simulink model "Boeing787_NewMission_ElectricalThermalHydraulicECS"  (R2016a)
settings: Solver=ode23tb  SolverMode=SingleTasking  StartTime=0.0  StopTime=346  RelTol=1e-3
InitFcn:
  | load('SampleOutput.mat')
  | 
  | load('SampleFuelBurn.mat')
undefined symbols (not defined in the file): ailerons, AirProp, B_737, CurrentMission, elevator, FuelBurn, HydProp, landing_gear, rudder, seed, thrust_rev
libraries: PowerFlowLib x68, simulink x20, powerlib_meascontrol x1
(part 14 of 24)

== system Boeing787_NewMission_ElectricalThermalHydraulicECS/Electrical/Generation Unit Sync-Sync4 ==
  engine speed : Inport
  battery voltage : Inport  Port=2
  idq0 : Inport  Port=3
  Temperature : Inport  Port=4
  Bus Creator : BusCreator  Inputs=3
  Bus Creator1 : BusCreator  Inputs=3
  Chopper (Averaged) : Subsystem  mask(Chopper.){}
      mask help: Basic chopper. Lossless storage elements. Switching model.
  Coeff of Resistance : Gain  Gain=3.85e-3
  Demux : Demux  Outputs=3
  Dot Product : DotProduct  InputSameDT=on  OutDataTypeStr=Inherit: Inherit via internal rule
  Exciter : Subsystem
      mask Display:
      | p = 0:0.1:(2*pi+0.1);
      | plot(sin(p), cos(p));
      | p1 = (-pi/8-0.1-0.2):0.1:(pi/8+0.1-0.2);
      | plot(0.8*sin(p1), 0.8*cos(p1), 0.8*sin(p1+pi), 0.8*cos(p1+pi));
      | p2 = sin((-pi/8-0.1-0.2+pi/8+0.1-0.2)/2);
      | p3 = sin((-pi/8-0.1-0.2+pi/8+0.1-0.2)/2+pi);
      | p4 = cos((-pi/8-0.1-0.2+pi/8+0.1-0.2)/2);
      | p5 = cos((-pi/8-0.1-0.2+pi/8+0.1-0.2)/2+pi);
      | plot(0.8*[p2, p3], 0.8*[p4, p5]);
      | port_label('output', 1, 'Vdq0');
      | port_label('output', 2, 'Te');
      | port_label('output', 3, 'Vfd');
      | port_label('output', 4, 'Ploss');
      | port_label('input', 1, 'idq0');
      | port_label('input', 2, 'w');
      | port_label('input', 3, 'ifd');
  Gain : Gain  Gain=200*2/3
  Gain1 : Gain  Gain=200
  Gain4 : Gain  Gain=0.001
  Gain5 : Gain  Gain=30
  Gain6 : Gain  Gain=0.02
  Generator : Subsystem
      mask Display:
      | p = 0:0.1:(2*pi+0.1);
      | plot(sin(p), cos(p));
      | p1 = (-pi/8-0.1-0.2):0.1:(pi/8+0.1-0.2);
      | plot(0.8*sin(p1), 0.8*cos(p1), 0.8*sin(p1+pi), 0.8*cos(p1+pi));
      | p2 = sin((-pi/8-0.1-0.2+pi/8+0.1-0.2)/2);
      | p3 = sin((-pi/8-0.1-0.2+pi/8+0.1-0.2)/2+pi);
      | p4 = cos((-pi/8-0.1-0.2+pi/8+0.1-0.2)/2);
      | p5 = cos((-pi/8-0.1-0.2+pi/8+0.1-0.2)/2+pi);
      | plot(0.8*[p2, p3], 0.8*[p4, p5]);
      | port_label('output', 1, 'Vdq0');
      | port_label('output', 2, 'Te');
      | port_label('output', 3, 'Vfd');
      | port_label('output', 4, 'Ploss');
      | port_label('input', 1, 'idq0');
      | port_label('input', 2, 'w');
      | port_label('input', 3, 'ifd');
  Initial Temperature : Constant  Value=25
  Integrator : Integrator  LimitOutput=on  UpperSaturationLimit=10  LowerSaturationLimit=-10
  Integrator1 : Integrator  LimitOutput=on  UpperSaturationLimit=1  LowerSaturationLimit=0
  RPM_to_radps : Gain  Gain=pi/30
  Sqrt : Sqrt  SaturateOnIntegerOverflow=on
  Sum : Sum  Inputs=++|
  Sum1 : Sum
  Sum2 : Sum  Inputs=+-|
  Sum3 : Sum  Inputs=-+|
  Sum4 : Sum  Inputs=+
  Sum5 : Sum  Inputs=|+-
  Sum6 : Sum  Inputs=|++
  Vcmd : Constant  Value=Vnom
  control1 : Constant
  data_sink : PowerFlowLib/Support Functions//Tools/data_sink
  one : Constant
  three-phase active rectifier Voltage Mode : PowerFlowLib/Energy & Power Systems/Electrical/Rectifiers/three-phase  active rectifier Voltage Mode  L=1  C=1e-4
  vdq0 : Outport
  battery current : Outport  Port=2
  engine torque : Outport  Port=3
  Ploss : Outport  Port=4
  wires:
  [R_temp_delta] -> Generator/4(Temp)
  [R_temp_delta] -> Exciter/4(Temp)
  [R_temp_delta] -> Chopper (Averaged)/3(Temperature)
  Sum6/1 -> [R_temp_delta]
  one/1 -> Sum6/2
  Coeff of Resistance/1 -> Sum6/1
  Sum5/1 -> Coeff of Resistance/1
  Initial Temperature/1 -> Sum5/2
  Temperature/1 -> Sum5/1
  engine speed/1 -> RPM_to_radps/1
  Bus Creator1/1 -> Bus Creator/1  "vdq0 (V)"
  Demux/3 -> Bus Creator1/3  "v0"
  Demux/2 -> Bus Creator1/2  "vq"
  Demux/1 -> Bus Creator1/1  "vd"
  Bus Creator/1 -> data_sink/1
  Sum/1 -> engine torque/1
  RPM_to_radps/1 -> Exciter/2(w), Generator/2(w)
  Exciter/1(vdq0) -> three-phase active rectifier Voltage Mode/1
  control1/1 -> three-phase active rectifier Voltage Mode/2
  Generator/3(vfd') -> Gain1/1
  Gain1/1 -> three-phase active rectifier Voltage Mode/3
  Gain/1 -> Bus Creator/3, Generator/3(ifd')  "Exciter current (A)"
  three-phase active rectifier Voltage Mode/1 -> Gain/1
  Exciter/2(Te) -> Sum/1
  Generator/2(Te) -> Sum/2
  idq0/1 -> Generator/1(idq0)
  Generator/1(vdq0) -> Demux/1, vdq0/1, Dot Product/2, Dot Product/1  "Vdq0 (V)"
  Chopper (Averaged)/1(iout) -> Exciter/3(ifd')
  battery voltage/1 -> Chopper (Averaged)/1(vin)
  Chopper (Averaged)/2(iin) -> battery current/1
  Exciter/4(Ploss) -> Sum1/1
  Generator/4(Ploss) -> Sum1/2
  Sum1/1 -> Ploss/1, Bus Creator/2  "Ploss (W)"
  Gain4/1 -> Integrator/1
  Sum2/1 -> Gain4/1
  Integrator/1 -> Sum3/2
  Sum3/1 -> Gain6/1
  Vcmd/1 -> Sum2/1
  Dot Product/1 -> Sum4/1
  Sum4/1 -> Sqrt/1
  Sqrt/1 -> Sum2/2
  Gain6/1 -> Integrator1/1
  Gain5/1 -> Sum3/1
  three-phase active rectifier Voltage Mode/2 -> Exciter/1(idq0)
  Integrator1/1 -> Chopper (Averaged)/2(q), Gain5/1

== system Boeing787_NewMission_ElectricalThermalHydraulicECS/Electrical/Generation Unit Sync-Sync5 ==
  engine speed : Inport
  battery voltage : Inport  Port=2
  idq0 : Inport  Port=3
  Temperature : Inport  Port=4
  Bus Creator : BusCreator  Inputs=3
  Bus Creator1 : BusCreator  Inputs=3
  Chopper (Averaged) : Subsystem  mask(Chopper.){}
      mask help: Basic chopper. Lossless storage elements. Switching model.
  Coeff of Resistance : Gain  Gain=3.85e-3
  Demux : Demux  Outputs=3
  Dot Product : DotProduct  InputSameDT=on  OutDataTypeStr=Inherit: Inherit via internal rule
  Exciter : Subsystem
      mask Display:
      | p = 0:0.1:(2*pi+0.1);
      | plot(sin(p), cos(p));
      | p1 = (-pi/8-0.1-0.2):0.1:(pi/8+0.1-0.2);
      | plot(0.8*sin(p1), 0.8*cos(p1), 0.8*sin(p1+pi), 0.8*cos(p1+pi));
      | p2 = sin((-pi/8-0.1-0.2+pi/8+0.1-0.2)/2);
      | p3 = sin((-pi/8-0.1-0.2+pi/8+0.1-0.2)/2+pi);
      | p4 = cos((-pi/8-0.1-0.2+pi/8+0.1-0.2)/2);
      | p5 = cos((-pi/8-0.1-0.2+pi/8+0.1-0.2)/2+pi);
      | plot(0.8*[p2, p3], 0.8*[p4, p5]);
      | port_label('output', 1, 'Vdq0');
      | port_label('output', 2, 'Te');
      | port_label('output', 3, 'Vfd');
      | port_label('output', 4, 'Ploss');
      | port_label('input', 1, 'idq0');
      | port_label('input', 2, 'w');
      | port_label('input', 3, 'ifd');
  Gain : Gain  Gain=200*2/3
  Gain1 : Gain  Gain=200
  Gain4 : Gain  Gain=0.001
  Gain5 : Gain  Gain=30
  Gain6 : Gain  Gain=0.02
  Generator : Subsystem
      mask Display:
      | p = 0:0.1:(2*pi+0.1);
      | plot(sin(p), cos(p));
      | p1 = (-pi/8-0.1-0.2):0.1:(pi/8+0.1-0.2);
      | plot(0.8*sin(p1), 0.8*cos(p1), 0.8*sin(p1+pi), 0.8*cos(p1+pi));
      | p2 = sin((-pi/8-0.1-0.2+pi/8+0.1-0.2)/2);
      | p3 = sin((-pi/8-0.1-0.2+pi/8+0.1-0.2)/2+pi);
      | p4 = cos((-pi/8-0.1-0.2+pi/8+0.1-0.2)/2);
      | p5 = cos((-pi/8-0.1-0.2+pi/8+0.1-0.2)/2+pi);
      | plot(0.8*[p2, p3], 0.8*[p4, p5]);
      | port_label('output', 1, 'Vdq0');
      | port_label('output', 2, 'Te');
      | port_label('output', 3, 'Vfd');
      | port_label('output', 4, 'Ploss');
      | port_label('input', 1, 'idq0');
      | port_label('input', 2, 'w');
      | port_label('input', 3, 'ifd');
  Initial Temperature : Constant  Value=25
  Integrator : Integrator  LimitOutput=on  UpperSaturationLimit=10  LowerSaturationLimit=-10
  Integrator1 : Integrator  LimitOutput=on  UpperSaturationLimit=1  LowerSaturationLimit=0
  RPM_to_radps : Gain  Gain=pi/30
  Sqrt : Sqrt  SaturateOnIntegerOverflow=on
  Sum : Sum  Inputs=++|
  Sum1 : Sum
  Sum2 : Sum  Inputs=+-|
  Sum3 : Sum  Inputs=-+|
  Sum4 : Sum  Inputs=+
  Sum5 : Sum  Inputs=|+-
  Sum6 : Sum  Inputs=|++
  Vcmd : Constant  Value=Vnom
  control1 : Constant
  data_sink : PowerFlowLib/Support Functions//Tools/data_sink
  one : Constant
  three-phase active rectifier Voltage Mode : PowerFlowLib/Energy & Power Systems/Electrical/Rectifiers/three-phase  active rectifier Voltage Mode  L=1  C=1e-4
  vdq0 : Outport
  battery current : Outport  Port=2
  engine torque : Outport  Port=3
  Ploss : Outport  Port=4
  wires:
  Integrator1/1 -> Gain5/1, Chopper (Averaged)/2(q)
  three-phase active rectifier Voltage Mode/2 -> Exciter/1(idq0)
  Gain5/1 -> Sum3/1
  Gain6/1 -> Integrator1/1
  Sqrt/1 -> Sum2/2
  Sum4/1 -> Sqrt/1
  Dot Product/1 -> Sum4/1
  Vcmd/1 -> Sum2/1
  Sum3/1 -> Gain6/1
  Integrator/1 -> Sum3/2
  Sum2/1 -> Gain4/1
  Gain4/1 -> Integrator/1
  Sum1/1 -> Bus Creator/2, Ploss/1  "Ploss (W)"
  Generator/4(Ploss) -> Sum1/2
  Exciter/4(Ploss) -> Sum1/1
  Chopper (Averaged)/2(iin) -> battery current/1
  battery voltage/1 -> Chopper (Averaged)/1(vin)
  Chopper (Averaged)/1(iout) -> Exciter/3(ifd')
  Generator/1(vdq0) -> Dot Product/1, Dot Product/2, vdq0/1, Demux/1  "Vdq0 (V)"
  idq0/1 -> Generator/1(idq0)
  Generator/2(Te) -> Sum/2
  Exciter/2(Te) -> Sum/1
  three-phase active rectifier Voltage Mode/1 -> Gain/1
  Gain/1 -> Generator/3(ifd'), Bus Creator/3  "Exciter current (A)"
  Gain1/1 -> three-phase active rectifier Voltage Mode/3
  Generator/3(vfd') -> Gain1/1
  control1/1 -> three-phase active rectifier Voltage Mode/2
  Exciter/1(vdq0) -> three-phase active rectifier Voltage Mode/1
  RPM_to_radps/1 -> Generator/2(w), Exciter/2(w)
  Sum/1 -> engine torque/1
  Bus Creator/1 -> data_sink/1
  Demux/1 -> Bus Creator1/1  "vd"
  Demux/2 -> Bus Creator1/2  "vq"
  Demux/3 -> Bus Creator1/3  "v0"
  Bus Creator1/1 -> Bus Creator/1  "vdq0 (V)"
  engine speed/1 -> RPM_to_radps/1
  Temperature/1 -> Sum5/1
  Initial Temperature/1 -> Sum5/2
  Sum5/1 -> Coeff of Resistance/1
  Coeff of Resistance/1 -> Sum6/1
  one/1 -> Sum6/2
  Sum6/1 -> [R_temp_delta]
  [R_temp_delta] -> Chopper (Averaged)/3(Temperature)
  [R_temp_delta] -> Exciter/4(Temp)
  [R_temp_delta] -> Generator/4(Temp)

== system Boeing787_NewMission_ElectricalThermalHydraulicECS/Electrical/Loads ==
  115VAC : Lookup_n-D  NumberOfTableDimensions=1  BreakpointsForDimension1=CurrentMission.tvec  Table=CurrentMission.V115ac  InterpMethod=Flat  InternalRulePriority=Speed  RndMeth=Simplest  InputSameDT=on
  230VAC : Lookup_n-D  NumberOfTableDimensions=1  BreakpointsForDimension1=CurrentMission.tvec  Table=CurrentMission.V230ac  InterpMethod=Flat  InternalRulePriority=Speed  RndMeth=Simplest  InputSameDT=on
  270VDC : Lookup_n-D  NumberOfTableDimensions=1  BreakpointsForDimension1=CurrentMission.tvec  Table=CurrentMission.V270dc  InterpMethod=Flat  InternalRulePriority=Speed  RndMeth=Simplest  InputSameDT=on
  28VDC : Lookup_n-D  NumberOfTableDimensions=1  BreakpointsForDimension1=CurrentMission.tvec  Table=CurrentMission.V28dc  InterpMethod=Flat  InternalRulePriority=Speed  RndMeth=Simplest  InputSameDT=on
  Clock : Clock
  Constant{,1..3} (4 alike) : Constant  Value=0
  Mux{,1..3} (4 alike) : Mux  Inputs=3
  PF{1..4} (4 alike) : Gain  Gain=0
  Product{,1..3} (4 alike) : Product
  Uniform Random Number : UniformRandomNumber  Minimum=0.95  Maximum=1.05  Seed=seed+500  SampleTime=1
  Uniform Random Number1 : UniformRandomNumber  Minimum=0.95  Maximum=1.05  Seed=seed  SampleTime=1
  Uniform Random Number2 : UniformRandomNumber  Minimum=0.95  Maximum=1.05  SampleTime=1
  Uniform Random Number3 : UniformRandomNumber  Minimum=0.95  Maximum=1.05  SampleTime=1
  kW to W{,1..3} (4 alike) : Gain  Gain=1000
  230 Vac Loads : Outport
  115 Vac Loads : Outport  Port=2
  270 Vdc Loads : Outport  Port=3
  28 Vdc Loads : Outport  Port=4
  wires:
  Mux2/1 -> 230 Vac Loads/1
  Mux/1 -> 270 Vdc Loads/1
  Clock/1 -> 28VDC/1, 270VDC/1, 115VAC/1, 230VAC/1
  PF3/1 -> Mux/2  "Q"
  270VDC/1 -> kW to W1/1  "P"
  PF2/1 -> Mux1/2  "Q"
  115VAC/1 -> kW to W2/1  "P"
  PF1/1 -> Mux2/2  "Q"
  230VAC/1 -> kW to W/1  "P"
  PF4/1 -> Mux3/2  "Q"
  28VDC/1 -> kW to W3/1  "P"
  Mux3/1 -> 28 Vdc Loads/1
  Constant/1 -> Mux/3
  Constant1/1 -> Mux3/3
  Constant2/1 -> Mux1/3
  Constant3/1 -> Mux2/3
  Mux1/1 -> 115 Vac Loads/1
  Product1/1 -> PF1/1, Mux2/1
  Product/1 -> PF2/1, Mux1/1
  Product2/1 -> PF3/1, Mux/1
  Product3/1 -> PF4/1, Mux3/1
  kW to W2/1 -> Product/2
  kW to W/1 -> Product1/2
  kW to W1/1 -> Product2/2
  kW to W3/1 -> Product3/2
  Uniform Random Number3/1 -> Product3/1
  Uniform Random Number2/1 -> Product2/1
  Uniform Random Number1/1 -> Product1/1
  Uniform Random Number/1 -> Product/1

== system Boeing787_NewMission_ElectricalThermalHydraulicECS/Electrical/Outputs ==
  Left_Wing_Toqrue_Nm : Inport
  Rght_Wing_Torque_Nm : Inport  Port=2
  APU_Torque_Nm : Inport  Port=3
  DC_Voltage_270 : Inport  Port=4
  Bus Creator : BusCreator  Inputs=4
  Electrical : Outport
  wires:
  Rght_Wing_Torque_Nm/1 -> Bus Creator/2  "Right Wing Torq (Nm)"
  APU_Torque_Nm/1 -> Bus Creator/3  "APU Torq (Nm)"
  Left_Wing_Toqrue_Nm/1 -> Bus Creator/1  "Left Wing Torq (Nm)"
  Bus Creator/1 -> Electrical/1
  DC_Voltage_270/1 -> Bus Creator/4  "DC_Voltage_270"

== system Boeing787_NewMission_ElectricalThermalHydraulicECS/Electrical/Thermal Interface ==
  Generator Loss [4] : Inport
  APU Loss [2] : Inport  Port=2
  Battery Loss [1] : Inport  Port=3
  Loadloss_W : Inport  Port=4
  Battery Thermal Model : Subsystem
  Constant{,1,3..4} (4 alike) : Constant  Value=0
  Constant2 : Constant  Value=25
  Constant5 : Constant  Value=25
  Coolant Temp : Constant  Value=25
  Coolant mdot : Constant  Value=0.5
  Demux : Demux
  Demux1 : Demux  Outputs=2
  Gain : Gain  Gain=50
  Generator 1 Thermal Model : Subsystem
  Generator 2 Thermal Model : Subsystem
  Generator 3 Thermal Model : Subsystem
  Generator 4 Thermal Model : Subsystem
  Generator 5 Thermal Model : Subsystem
  Generator 6 Thermal Model : Subsystem
  Load Thermal Model : Subsystem
  Mux : Mux
  To Workspace6 : ToWorkspace  VariableName=gen_temps  SaveFormat=Structure With Time  SampleTime=-1
  air Temp : Constant  Value=25
  Tgen1 : Outport
  Tgen2 : Outport  Port=2
  Tgen3 : Outport  Port=3
  Tgen4 : Outport  Port=4
  Tgen5 : Outport  Port=5
  Tgen6 : Outport  Port=6
  Tbatt : Outport  Port=7
  TLoad : Outport  Port=8
  wires:
  Generator Loss [4]/1 -> Gain/1
  Demux/1 -> Generator 1 Thermal Model/1(Ploss)
  Demux/2 -> Generator 2 Thermal Model/1(Ploss)
  Demux/3 -> Generator 3 Thermal Model/1(Ploss)
  Demux/4 -> Generator 4 Thermal Model/1(Ploss)
  Generator 4 Thermal Model/1(T_gen) -> Mux/4, Tgen4/1
  Generator 2 Thermal Model/1(T_gen) -> Mux/2, Tgen2/1
  Generator 1 Thermal Model/1(T_gen) -> Mux/1, Tgen1/1
  APU Loss [2]/1 -> Demux1/1
  Demux1/1 -> Generator 5 Thermal Model/1(Ploss)
  Demux1/2 -> Generator 6 Thermal Model/1(Ploss)
  Generator 6 Thermal Model/1(T_gen) -> Tgen6/1
  Generator 5 Thermal Model/1(T_gen) -> Tgen5/1
  Coolant Temp/1 -> [Tf]
  air Temp/1 -> [Ta]
  Coolant mdot/1 -> [mdot]
  [mdot] -> Generator 1 Thermal Model/4(coolant mdot)
  [Tf] -> Generator 1 Thermal Model/2(Liquid Coolant Temp)
  [Ta] -> Generator 1 Thermal Model/3(Air Temp)
  [Tf] -> Generator 6 Thermal Model/2(Liquid Coolant Temp)
  [Ta] -> Generator 6 Thermal Model/3(Air Temp)
  [mdot] -> Generator 6 Thermal Model/4(coolant mdot)
  [Tf] -> Generator 5 Thermal Model/2(Liquid Coolant Temp)
  [Ta] -> Generator 5 Thermal Model/3(Air Temp)
  [mdot] -> Generator 5 Thermal Model/4(coolant mdot)
  [mdot] -> Generator 4 Thermal Model/4(coolant mdot)
  [Ta] -> Generator 4 Thermal Model/3(Air Temp)
  [Tf] -> Generator 4 Thermal Model/2(Liquid Coolant Temp)
  [Tf] -> Generator 3 Thermal Model/2(Liquid Coolant Temp)
  [Ta] -> Generator 3 Thermal Model/3(Air Temp)
  [mdot] -> Generator 3 Thermal Model/4(coolant mdot)
  [Tf] -> Generator 2 Thermal Model/2(Liquid Coolant Temp)
  [mdot] -> Generator 2 Thermal Model/4(coolant mdot)
  [Ta] -> Generator 2 Thermal Model/3(Air Temp)
  Battery Loss [1]/1 -> Battery Thermal Model/1(Ploss)
  Loadloss_W/1 -> Load Thermal Model/1(Ploss)
  Constant/1 -> Battery Thermal Model/2(Liquid Coolant Temp)
  Constant1/1 -> Battery Thermal Model/4(coolant mdot)
  Constant2/1 -> Battery Thermal Model/3(Air Temp)
  Constant4/1 -> Load Thermal Model/4(coolant mdot)
  Constant3/1 -> Load Thermal Model/2(Liquid Coolant Temp)
  Constant5/1 -> Load Thermal Model/3(Air Temp)
  Battery Thermal Model/1(T_Batt) -> Tbatt/1
  Load Thermal Model/1(T_gen) -> TLoad/1
  Generator 3 Thermal Model/1(T_gen) -> Mux/3, Tgen3/1
  Mux/1 -> To Workspace6/1
  Gain/1 -> Demux/1

== system Boeing787_NewMission_ElectricalThermalHydraulicECS/Electrical/Transformer-rectifier ==
  vqd0 : Inport
  iDC : Inport  Port=2
  Constant1 : Constant  Value=270
  Constant2 : Constant  Value=1.0
  Control : Subsystem
  Sum1 : Sum  Inputs=|++
  Three-phase Full Bridge Rectifier : Subsystem  AncestorBlock=PowerFlowLib/Energy & Power Systems/Electrical/Rectifiers/Three-phase Full Bridge1  mask(Single-phase full bridge rectifier.){C=100e-6, Rc=1}
      mask prompts: C "Output capacitance (F):"; Rc "Circuit parasitic resistance (ohm):"
      mask help: Single-phase Full bridge rectifier. Lead resistance is added to make simulation possible.
  Transformer1 : Subsystem  AncestorBlock=PowerFlowLib/Energy & Power Systems/Electrical/Machines/Transformer  mask(Transformer){Rp=0.005, Rs=0.1, N1=400, N2=332*1.4}
      mask prompts: Rp "Primary Winding Resistance"; Rs "Secondary Winding Resistance"; N1 "Number of Turns in Primary"; N2 "Number of Turns in Secondary"
      mask help:
      | The user inputs and outputs are given below. Inputs to the model are:
      |
      | Block Inputs
      | #1: Primary voltage input [V]
      | #2: Secondary current input [A]
      |
      | Block Outputs
      | #1: Secondary voltage output [V]
      | #2: Primary current input [A]
      mask Help: eval('open(''Transformer Help.html'')');
      mask Display:
      | image(imread('Transformer.png'))
      | 
      | port_label('input',1,'{\bf V_i_n}','TexMode','on')
      | port_label('input',2,'{\bf I_o_u_t}','TexMode','on')
      | 
      | port_label('output',1,'{\bf V_o_u_t}','TexMode','on')
      | port_label('output',2,'{\bf I_i_n}','TexMode','on')
  vout : Outport
  iqd0 : Outport  Port=2
  wires:
  Transformer1/2(Iin) -> iqd0/1
  Transformer1/1(Vout) -> Three-phase Full Bridge Rectifier/2(vin)
  vqd0/1 -> Transformer1/1(Vin)
  Three-phase Full Bridge Rectifier/2(iin) -> Transformer1/2(Iout)
  iDC/1 -> Three-phase Full Bridge Rectifier/1(iout)
  Three-phase Full Bridge Rectifier/1(vout) -> Control/1(Vout), vout/1
  Constant1/1 -> Control/2(ref)
  Constant2/1 -> Sum1/1
  Control/1(u) -> Sum1/2
  Sum1/1 -> Three-phase Full Bridge Rectifier/3(u)

== system Boeing787_NewMission_ElectricalThermalHydraulicECS/Electrical/Transformer-rectifier1 ==
  vqd0 : Inport
  iDC : Inport  Port=2
  Constant : Constant
  Constant1 : Constant  Value=28
  Control : Subsystem
  Saturation : Saturate  UpperLimit=inf  LowerLimit=-inf
  Sum1 : Sum  Inputs=|++
  Three-phase Full Bridge1 : Subsystem  AncestorBlock=PowerFlowLib/Energy & Power Systems/Electrical/Rectifiers/Three-phase Full Bridge1  mask(Single-phase full bridge rectifier.){C=100e-6, Rc=1}
      mask prompts: C "Output capacitance (F):"; Rc "Circuit parasitic resistance (ohm):"
      mask help: Single-phase Full bridge rectifier. Lead resistance is added to make simulation possible.
  Transformer1 : Subsystem  AncestorBlock=PowerFlowLib/Energy & Power Systems/Electrical/Machines/Transformer  mask(Transformer){Rp=0.005, Rs=0.1, N1=400, N2=45}
      mask prompts: Rp "Primary Winding Resistance"; Rs "Secondary Winding Resistance"; N1 "Number of Turns in Primary"; N2 "Number of Turns in Secondary"
      mask help:
      | The user inputs and outputs are given below. Inputs to the model are:
      |
      | Block Inputs
      | #1: Primary voltage input [V]
      | #2: Secondary current input [A]
      |
      | Block Outputs
      | #1: Secondary voltage output [V]
      | #2: Primary current input [A]
      mask Help: eval('open(''Transformer Help.html'')');
      mask Display:
      | image(imread('Transformer.png'))
      | 
      | port_label('input',1,'{\bf V_i_n}','TexMode','on')
      | port_label('input',2,'{\bf I_o_u_t}','TexMode','on')
      | 
      | port_label('output',1,'{\bf V_o_u_t}','TexMode','on')
      | port_label('output',2,'{\bf I_i_n}','TexMode','on')
  vout : Outport
  iqd0 : Outport  Port=2
  wires:
  Three-phase Full Bridge1/1(vout) -> Control/1(Vout), vout/1
  iDC/1 -> Three-phase Full Bridge1/1(iout)
  Three-phase Full Bridge1/2(iin) -> Transformer1/2(Iout)
  vqd0/1 -> Transformer1/1(Vin)
  Transformer1/1(Vout) -> Three-phase Full Bridge1/2(vin)
  Transformer1/2(Iin) -> iqd0/1
  Constant1/1 -> Control/2(ref)
  Constant/1 -> Sum1/1
  Control/1(u) -> Sum1/2
  Sum1/1 -> Saturation/1
  Saturation/1 -> Three-phase Full Bridge1/3(u)

== system Boeing787_NewMission_ElectricalThermalHydraulicECS/Eng1/Gearbox ==
  w_engine : Inport
  T_gen : Inport  Port=2
  1-tran_efficiency : Gain  Gain=1-Gear_Efficiency/100  SaturateOnIntegerOverflow=on  OutDataTypeStr=Inherit: Same as input  ParamDataTypeStr=Inherit: Same as input
  Gain : Gain  Gain=Gear_Ratio
  Gain1 : Gain  Gain=Gear_Ratio
  Memory1 : Memory
  Sum : Sum  Inputs=-++  SaturateOnIntegerOverflow=on  InputSameDT=on  OutDataTypeStr=Inherit: Same as first input
  gear1 NL loss : Lookup  InputValues=[0;1000;2000;3000;4000;5000;6000]*2*pi/60  Table=[0;0.735;1.334;1.491;1.525;1.212;1.276]  SaturateOnIntegerOverflow=on
  tran_efficiency : Gain  Gain=Gear_Efficiency/4/100  SaturateOnIntegerOverflow=on  OutDataTypeStr=Inherit: Same as input  ParamDataTypeStr=Inherit: Same as input
  w_shaft : Outport
  T_shaft : Outport  Port=2
  wires:
  Gain/1 -> w_shaft/1
  Gain1/1 -> Memory1/1
  T_gen/1 -> Gain1/1, 1-tran_efficiency/1
  w_engine/1 -> Gain/1, gear1 NL loss/1
  gear1 NL loss/1 -> tran_efficiency/1
  Memory1/1 -> Sum/3
  1-tran_efficiency/1 -> Sum/2
  tran_efficiency/1 -> Sum/1
  Sum/1 -> T_shaft/1

== system Boeing787_NewMission_ElectricalThermalHydraulicECS/Eng1/Unit Conversion  ==
  Signal_in : Inport
  conv_fcn : Fcn  Expr=u(1)/745.69987
  Converted Signal Out : Outport
  wires:
  Signal_in/1 -> conv_fcn/1
  conv_fcn/1 -> Converted Signal Out/1

== system Boeing787_NewMission_ElectricalThermalHydraulicECS/Eng1/Unit Conversion 1 ==
  Signal_in : Inport
  conv_fcn : Fcn  Expr=u(1)/1.8
  Converted Signal Out : Outport
  wires:
  conv_fcn/1 -> Converted Signal Out/1
  Signal_in/1 -> conv_fcn/1

== system Boeing787_NewMission_ElectricalThermalHydraulicECS/Eng1/Unit Conversion 4 ==
  Signal_in : Inport
  conv_fcn : Fcn  Expr=u(1)/(1.450377e-1)
  Converted Signal Out : Outport
  wires:
  Signal_in/1 -> conv_fcn/1
  conv_fcn/1 -> Converted Signal Out/1

== system Boeing787_NewMission_ElectricalThermalHydraulicECS/Eng1/Unit Conversion 5 ==
  Signal_in : Inport
  conv_fcn : Fcn  Expr=u(1)*.45359237
  Converted Signal Out : Outport
  wires:
  Signal_in/1 -> conv_fcn/1
  conv_fcn/1 -> Converted Signal Out/1

== system Boeing787_NewMission_ElectricalThermalHydraulicECS/Eng2/Gearbox ==
  w_engine : Inport
  T_gen : Inport  Port=2
  1-tran_efficiency : Gain  Gain=1-Gear_Efficiency/100  SaturateOnIntegerOverflow=on  OutDataTypeStr=Inherit: Same as input  ParamDataTypeStr=Inherit: Same as input
  Gain : Gain  Gain=Gear_Ratio
  Gain1 : Gain  Gain=Gear_Ratio
  Memory1 : Memory
  Sum : Sum  Inputs=-++  SaturateOnIntegerOverflow=on  InputSameDT=on  OutDataTypeStr=Inherit: Same as first input
  gear1 NL loss : Lookup  InputValues=[0;1000;2000;3000;4000;5000;6000]*2*pi/60  Table=[0;0.735;1.334;1.491;1.525;1.212;1.276]  SaturateOnIntegerOverflow=on
  tran_efficiency : Gain  Gain=Gear_Efficiency/4/100  SaturateOnIntegerOverflow=on  OutDataTypeStr=Inherit: Same as input  ParamDataTypeStr=Inherit: Same as input
  w_shaft : Outport
  T_shaft : Outport  Port=2
  wires:
  Sum/1 -> T_shaft/1
  tran_efficiency/1 -> Sum/1
  1-tran_efficiency/1 -> Sum/2
  Memory1/1 -> Sum/3
  gear1 NL loss/1 -> tran_efficiency/1
  w_engine/1 -> gear1 NL loss/1, Gain/1
  T_gen/1 -> 1-tran_efficiency/1, Gain1/1
  Gain1/1 -> Memory1/1
  Gain/1 -> w_shaft/1

== system Boeing787_NewMission_ElectricalThermalHydraulicECS/Eng2/Unit Conversion  ==
  Signal_in : Inport
  conv_fcn : Fcn  Expr=u(1)/745.69987
  Converted Signal Out : Outport
  wires:
  conv_fcn/1 -> Converted Signal Out/1
  Signal_in/1 -> conv_fcn/1

== system Boeing787_NewMission_ElectricalThermalHydraulicECS/Eng2/Unit Conversion 1 ==
  Signal_in : Inport
  conv_fcn : Fcn  Expr=u(1)/1.8
  Converted Signal Out : Outport
  wires:
  Signal_in/1 -> conv_fcn/1
  conv_fcn/1 -> Converted Signal Out/1

== system Boeing787_NewMission_ElectricalThermalHydraulicECS/Eng2/Unit Conversion 4 ==
  Signal_in : Inport
  conv_fcn : Fcn  Expr=u(1)/(1.450377e-1)
  Converted Signal Out : Outport
  wires:
  conv_fcn/1 -> Converted Signal Out/1
  Signal_in/1 -> conv_fcn/1

== system Boeing787_NewMission_ElectricalThermalHydraulicECS/Eng2/Unit Conversion 5 ==
  Signal_in : Inport
  conv_fcn : Fcn  Expr=u(1)*.45359237
  Converted Signal Out : Outport
  wires:
  conv_fcn/1 -> Converted Signal Out/1
  Signal_in/1 -> conv_fcn/1

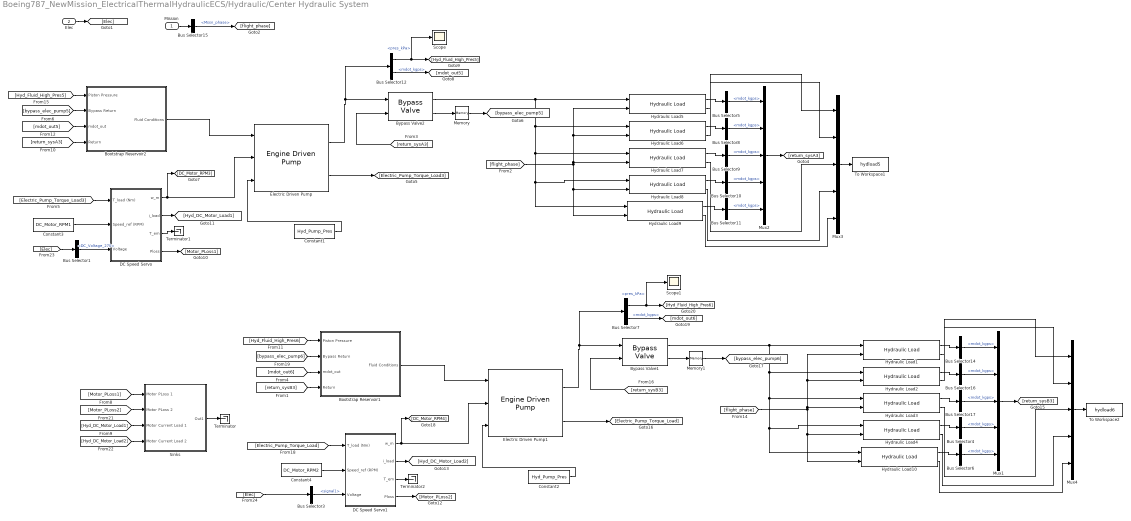
== system Boeing787_NewMission_ElectricalThermalHydraulicECS/Hydraulic/Center Hydraulic System ==
  Mission : Inport
  Elec : Inport  Port=2
  Bootstrap Reservoir1 : Subsystem  mask(Fluid Reservoir){res_vol=.25, High_Pres_Area=.05, Low_Pres_Area=0, pres_loss=1, T_init=300, P_init=1500, mass_init=30}
      mask prompts: res_vol "Resevoir Volume [m³]"; High_Pres_Area "High Pressure Piston Area"; Low_Pres_Area "Low Pressure Piston Area"; pres_loss "Air Pressure Losses [%]"; T_init "Initial Fluid Temp [K]"; P_init "Initial Air Pressure [kPa]"; mass_init "Initial Fluid Mass [kg]"
      mask help:
      | The fluid reservoir serves as a tank for storing excess hydraulic fluid.
      | The reservoir is fed by returning hydraulic fluid and feeds the engine driven pump.
      | Currently the fluid reservoir tracks the time dependent mass and temperature of the hydraulic fluid in the tank.
      |
      | Block Inputs
      | #1: Bleed air properties (Bus signal)
      | #2: Bypass return from bypass valve
      | #3: Mass flow rate pumped out by hydraulic pump
      | #4: Mass flow rate returned from actuators
      |
      | Block Outputs
      | #1: Bleed air demanded to maintain pressurization
      | #2: Hydraulic fluid properties in the reservoir
      mask init:
      | load AirProp
      | load HydProp
      mask Help: eval('open(''FluidReservoir_help.html'')');
      mask Display:
      | image(imread('hyd_res.png'))
      | 
      | port_label('input',1,'{\bf High Piston Pressure}','TexMode','on')
      | port_label('input',2,'{\bf Bypass Return}','TexMode','on')
      | port_label('input',3,'{\bf m_d_o_t Out}','TexMode','on')
      | port_label('input',4,'{\bf m_d_o_t Return}','TexMode','on')
      | 
      | 
      | port_label('output',1,'{\bf Fluid Out}','TexMode','on')
  Bootstrap Reservoir2 : Subsystem  mask(Fluid Reservoir){res_vol=.25, High_Pres_Area=.05, Low_Pres_Area=0, pres_loss=1, T_init=300, P_init=1500, mass_init=30}
      mask prompts: res_vol "Resevoir Volume [m³]"; High_Pres_Area "High Pressure Piston Area"; Low_Pres_Area "Low Pressure Piston Area"; pres_loss "Air Pressure Losses [%]"; T_init "Initial Fluid Temp [K]"; P_init "Initial Air Pressure [kPa]"; mass_init "Initial Fluid Mass [kg]"
      mask help:
      | The fluid reservoir serves as a tank for storing excess hydraulic fluid.
      | The reservoir is fed by returning hydraulic fluid and feeds the engine driven pump.
      | Currently the fluid reservoir tracks the time dependent mass and temperature of the hydraulic fluid in the tank.
      |
      | Block Inputs
      | #1: Bleed air properties (Bus signal)
      | #2: Bypass return from bypass valve
      | #3: Mass flow rate pumped out by hydraulic pump
      | #4: Mass flow rate returned from actuators
      |
      | Block Outputs
      | #1: Bleed air demanded to maintain pressurization
      | #2: Hydraulic fluid properties in the reservoir
      mask init:
      | load AirProp
      | load HydProp
      mask Help: eval('open(''FluidReservoir_help.html'')');
      mask Display:
      | image(imread('hyd_res.png'))
      | 
      | port_label('input',1,'{\bf High Piston Pressure}','TexMode','on')
      | port_label('input',2,'{\bf Bypass Return}','TexMode','on')
      | port_label('input',3,'{\bf m_d_o_t Out}','TexMode','on')
      | port_label('input',4,'{\bf m_d_o_t Return}','TexMode','on')
      | 
      | 
      | port_label('output',1,'{\bf Fluid Out}','TexMode','on')
  Bus Selector1 : BusSelector  OutputSignals=signal1.DC_Voltage_270
  Bus Selector{4..6,8..11,14,16..17} (10 alike) : BusSelector  OutputSignals=mdot_kgps
  Bus Selector12 : BusSelector  OutputSignals=pres_kPa,mdot_kgps
  Bus Selector15 : BusSelector  OutputSignals=Mssn_phase
  Bus Selector3 : BusSelector  OutputSignals=signal1
  Bus Selector7 : BusSelector  OutputSignals=pres_kPa,mdot_kgps
  Bypass Valve1 : PowerFlowLib/Energy & Power Systems/Hydraulic/Bypass Valve
  Bypass Valve2 : PowerFlowLib/Energy & Power Systems/Hydraulic/Bypass Valve
  Constant1 : Constant  Value=Hyd_Pump_Pres
  Constant2 : Constant  Value=Hyd_Pump_Pres
  Constant3 : Constant  Value=DC_Motor_RPM1
  Constant4 : Constant  Value=DC_Motor_RPM2
  DC Speed Servo : Subsystem  AncestorBlock=PowerFlowLib/Energy & Power Systems/Electrical/Machines/DC Speed Servo  mask{Vf=390, Ra=0.05, La=0.9e-3, Rfsh=400, Lfsh=320, Lmsh=1.9, J=1.5}
      mask prompts: Vf "Field voltage (V)"; Ra "Armature resistance (Ohms)"; La "Armature inductance (H)"; Rfsh "Shunt field resistance (Ohms)"; Lfsh "Shunt field inductance (H)"; Lmsh "Mutual inductance (H)"; J "Rotor moment of inertia (Kgm^2)"
  DC Speed Servo1 : Subsystem  AncestorBlock=PowerFlowLib/Energy & Power Systems/Electrical/Machines/DC Speed Servo  mask{Vf=390, Ra=0.05, La=0.9e-3, Rfsh=400, Lfsh=320, Lmsh=1.9, J=1.5}
      mask prompts: Vf "Field voltage (V)"; Ra "Armature resistance (Ohms)"; La "Armature inductance (H)"; Rfsh "Shunt field resistance (Ohms)"; Lfsh "Shunt field inductance (H)"; Lmsh "Mutual inductance (H)"; J "Rotor moment of inertia (Kgm^2)"
  Electric Driven Pump : PowerFlowLib/Energy & Power Systems/Hydraulic/Engine Driven Pump  RPM=3750  disp=39  eta_mech=95  eta_v=85  nom_T=40  nom_w=393  nom_delP=20684
  Electric Driven Pump1 : PowerFlowLib/Energy & Power Systems/Hydraulic/Engine Driven Pump  RPM=3750  disp=39  eta_mech=95  eta_v=85  nom_T=40  nom_w=393  nom_delP=20684
  Hydraulic Load1 : PowerFlowLib/Energy & Power Systems/Hydraulic/Hydraulic Load  fileslct=off  filename=HydraulicLoad.mat  filedir=C:\Users\mwillms4\Dropbox\School\Graduate\Research\PowerFlow Development\PowerFlow Summer 2013\PropertyTables\HydraulicLoad.mat  var_struct=HydraulicLoad  h_load=B_737 - rudder
  Hydraulic Load10 : PowerFlowLib/Energy & Power Systems/Hydraulic/Hydraulic Load  fileslct=off  filename=HydraulicLoad.mat  filedir=C:\Users\mwillms4\Dropbox\School\Graduate\Research\PowerFlow Development\PowerFlow Summer 2013\PropertyTables\HydraulicLoad.mat  var_struct=HydraulicLoad  h_load=B_737 - thrust_rev
  Hydraulic Load2 : PowerFlowLib/Energy & Power Systems/Hydraulic/Hydraulic Load  fileslct=off  filename=HydraulicLoad.mat  filedir=C:\Users\mwillms4\Dropbox\School\Graduate\Research\PowerFlow Development\PowerFlow Summer 2013\PropertyTables\HydraulicLoad.mat  var_struct=HydraulicLoad  h_load=B_737 - ailerons
  Hydraulic Load3 : PowerFlowLib/Energy & Power Systems/Hydraulic/Hydraulic Load  fileslct=off  filename=HydraulicLoad.mat  filedir=C:\Users\mwillms4\Dropbox\School\Graduate\Research\PowerFlow Development\PowerFlow Summer 2013\PropertyTables\HydraulicLoad.mat  var_struct=HydraulicLoad  h_load=B_737 - elevator
  Hydraulic Load4 : PowerFlowLib/Energy & Power Systems/Hydraulic/Hydraulic Load  fileslct=off  filename=HydraulicLoad.mat  filedir=C:\Users\mwillms4\Dropbox\School\Graduate\Research\PowerFlow Development\PowerFlow Summer 2013\PropertyTables\HydraulicLoad.mat  var_struct=HydraulicLoad  h_load=B_737 - landing_gear
  Hydraulic Load5 : PowerFlowLib/Energy & Power Systems/Hydraulic/Hydraulic Load  fileslct=off  filename=HydraulicLoad.mat  filedir=C:\Users\mwillms4\Dropbox\School\Graduate\Research\PowerFlow Development\PowerFlow Summer 2013\PropertyTables\HydraulicLoad.mat  var_struct=HydraulicLoad  h_load=B_737 - rudder
  Hydraulic Load6 : PowerFlowLib/Energy & Power Systems/Hydraulic/Hydraulic Load  fileslct=off  filename=HydraulicLoad.mat  filedir=C:\Users\mwillms4\Dropbox\School\Graduate\Research\PowerFlow Development\PowerFlow Summer 2013\PropertyTables\HydraulicLoad.mat  var_struct=HydraulicLoad  h_load=B_737 - ailerons
  Hydraulic Load7 : PowerFlowLib/Energy & Power Systems/Hydraulic/Hydraulic Load  fileslct=off  filename=HydraulicLoad.mat  filedir=C:\Users\mwillms4\Dropbox\School\Graduate\Research\PowerFlow Development\PowerFlow Summer 2013\PropertyTables\HydraulicLoad.mat  var_struct=HydraulicLoad  h_load=B_737 - elevator
  Hydraulic Load8 : PowerFlowLib/Energy & Power Systems/Hydraulic/Hydraulic Load  fileslct=off  filename=HydraulicLoad.mat  filedir=C:\Users\mwillms4\Dropbox\School\Graduate\Research\PowerFlow Development\PowerFlow Summer 2013\PropertyTables\HydraulicLoad.mat  var_struct=HydraulicLoad  h_load=B_737 - landing_gear
  Hydraulic Load9 : PowerFlowLib/Energy & Power Systems/Hydraulic/Hydraulic Load  fileslct=off  filename=HydraulicLoad.mat  filedir=C:\Users\mwillms4\Dropbox\School\Graduate\Research\PowerFlow Development\PowerFlow Summer 2013\PropertyTables\HydraulicLoad.mat  var_struct=HydraulicLoad  h_load=B_737 - thrust_rev
  Memory : Memory
  Memory1 : Memory
  Mux{1..4} (4 alike) : Mux  Inputs=5
  Scope : Scope
  Scope1 : Scope
  Sinks : Subsystem
  Terminator : Terminator
  Terminator1 : Terminator
  Terminator2 : Terminator
  To Workspace1 : ToWorkspace  VariableName=hydload5  SaveFormat=Structure With Time  SampleTime=10
  To Workspace2 : ToWorkspace  VariableName=hydload6  SaveFormat=Structure With Time  SampleTime=10
  wires:
  Bus Selector15/1 -> [flight_phase]  "<Mssn_phase>"
  Mission/1 -> Bus Selector15/1
  DC Speed Servo/1(w_m) -> Electric Driven Pump/2, [DC_Motor_RPM3]
  Bus Selector1/1 -> DC Speed Servo/3(Voltage)  "<DC_Voltage_270>"
  Hydraulic Load5/1 -> Bus Selector5/1
  Bypass Valve2/1 -> Hydraulic Load9/1, Hydraulic Load8/1, Hydraulic Load7/1, Hydraulic Load6/1, Hydraulic Load5/1
  Hydraulic Load6/2 -> Mux3/2
  Hydraulic Load7/2 -> Mux3/3
  Hydraulic Load6/1 -> Bus Selector8/1
  Hydraulic Load7/1 -> Bus Selector9/1
  Bus Selector8/1 -> Mux2/2  "<mdot_kgps>"
  Bus Selector5/1 -> Mux2/1  "<mdot_kgps>"
  Bus Selector9/1 -> Mux2/3  "<mdot_kgps>"
  Mux2/1 -> [return_sysA3]
  [flight_phase] -> Hydraulic Load9/2, Hydraulic Load8/2, Hydraulic Load5/2, Hydraulic Load6/2, Hydraulic Load7/2
  Hydraulic Load8/1 -> Bus Selector10/1
  Hydraulic Load9/1 -> Bus Selector11/1
  Hydraulic Load9/2 -> Mux3/5
  Hydraulic Load8/2 -> Mux3/4
  Bus Selector10/1 -> Mux2/4  "<mdot_kgps>"
  Bus Selector11/1 -> Mux2/5  "<mdot_kgps>"
  Hydraulic Load5/2 -> Mux3/1
  Mux3/1 -> To Workspace1/1
  Electric Driven Pump/1 -> Bus Selector12/1, Bypass Valve2/1
  [return_sysA3] -> Bypass Valve2/2
  Constant1/1 -> Electric Driven Pump/3
  Electric Driven Pump/2 -> [Electric_Pump_Torque_Load3]
  [Electric_Pump_Torque_Load3] -> DC Speed Servo/1(T_load (Nm))
  Bypass Valve2/2 -> Memory/1
  [bypass_elec_pump5] -> Bootstrap Reservoir2/2(Bypass Return)
  Bootstrap Reservoir2/1(Fluid Conditions) -> Electric Driven Pump/1
  Constant3/1 -> DC Speed Servo/2(Speed_ref (RPM))
  Bus Selector12/1 -> Scope/1, [Hyd_Fluid_High_Pres5]  "<pres_kPa>"
  Bus Selector12/2 -> [mdot_out5]  "<mdot_kgps>"
  DC Speed Servo/4(Ploss) -> [Motor_PLoss1]
  [Motor_PLoss1] -> Sinks/1("Motor PLoss 1 ")
  DC Speed Servo/2(i_load) -> [Hyd_DC_Motor_Load1]
  [Hyd_DC_Motor_Load1] -> Sinks/3(Motor Current Load 1)
  [return_sysA3] -> Bootstrap Reservoir2/4(Return)
  [mdot_out5] -> Bootstrap Reservoir2/3(mdot_out)
  [Hyd_Fluid_High_Pres5] -> Bootstrap Reservoir2/1(Piston Pressure)
  DC Speed Servo1/1(w_m) -> Electric Driven Pump1/2, [DC_Motor_RPM4]
  [Elec] -> Bus Selector3/1
  Bus Selector3/1 -> DC Speed Servo1/3(Voltage)  "<signal1>"
  Hydraulic Load1/1 -> Bus Selector14/1
  Bypass Valve1/1 -> Hydraulic Load10/1, Hydraulic Load4/1, Hydraulic Load3/1, Hydraulic Load2/1, Hydraulic Load1/1
  Hydraulic Load2/2 -> Mux4/2
  Hydraulic Load3/2 -> Mux4/3
  Hydraulic Load2/1 -> Bus Selector16/1
  Hydraulic Load3/1 -> Bus Selector17/1
  Bus Selector16/1 -> Mux1/2  "<mdot_kgps>"
  Bus Selector14/1 -> Mux1/1  "<mdot_kgps>"
  Bus Selector17/1 -> Mux1/3  "<mdot_kgps>"
  Mux1/1 -> [return_sysB3]
  [flight_phase] -> Hydraulic Load10/2, Hydraulic Load4/2, Hydraulic Load1/2, Hydraulic Load2/2, Hydraulic Load3/2
  Hydraulic Load4/1 -> Bus Selector4/1
  Hydraulic Load10/1 -> Bus Selector6/1
  Hydraulic Load10/2 -> Mux4/5
  Hydraulic Load4/2 -> Mux4/4
  Bus Selector4/1 -> Mux1/4  "<mdot_kgps>"
  Bus Selector6/1 -> Mux1/5  "<mdot_kgps>"
  Hydraulic Load1/2 -> Mux4/1
  Mux4/1 -> To Workspace2/1
  Electric Driven Pump1/1 -> Bus Selector7/1, Bypass Valve1/1
  [return_sysB3] -> Bypass Valve1/2
  Constant2/1 -> Electric Driven Pump1/3
  Electric Driven Pump1/2 -> [Electric_Pump_Torque_Load]
  [Electric_Pump_Torque_Load] -> DC Speed Servo1/1(T_load (Nm))
  Bypass Valve1/2 -> Memory1/1
  [bypass_elec_pump6] -> Bootstrap Reservoir1/2(Bypass Return)
  Bootstrap Reservoir1/1(Fluid Conditions) -> Electric Driven Pump1/1
  Constant4/1 -> DC Speed Servo1/2(Speed_ref (RPM))
  Bus Selector7/1 -> Scope1/1, [Hyd_Fluid_High_Pres6]  "<pres_kPa>"
  Bus Selector7/2 -> [mdot_out6]  "<mdot_kgps>"
  DC Speed Servo1/4(Ploss) -> [Motor_PLoss2]
  DC Speed Servo1/2(i_load) -> [Hyd_DC_Motor_Load2]
  [return_sysB3] -> Bootstrap Reservoir1/4(Return)
  [mdot_out6] -> Bootstrap Reservoir1/3(mdot_out)
  [Hyd_Fluid_High_Pres6] -> Bootstrap Reservoir1/1(Piston Pressure)
  [Motor_PLoss2] -> Sinks/2(Motor PLoss 2)
  [Hyd_DC_Motor_Load2] -> Sinks/4(Motor Current Load 2)
  [Elec] -> Bus Selector1/1
  Elec/1 -> [Elec]
  Sinks/1(Out1) -> Terminator/1
  DC Speed Servo1/3(T_em) -> Terminator2/1
  DC Speed Servo/3(T_em) -> Terminator1/1
  Memory/1 -> [bypass_elec_pump5]
  Memory1/1 -> [bypass_elec_pump6]
